simulink model "Ejemplo_1"  (R2022a)
settings: Solver=ode4  StartTime=0.0  StopTime=10.0  FixedStep=0.001  RelTol=1e-3
settings Model: Creator=Anahi Monserrat  LastModifiedBy=Anahi Monserrat

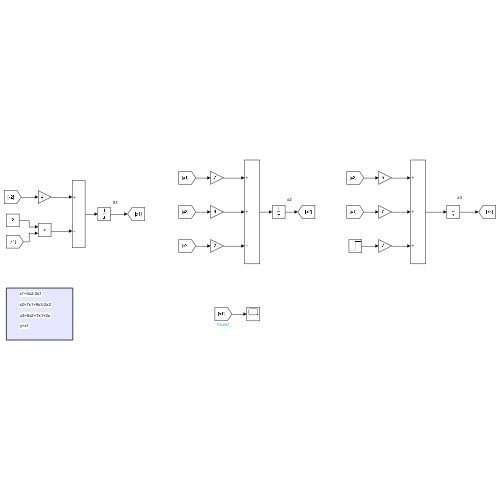
[thumbnail: Simulink's stored preview of the top-level diagram]
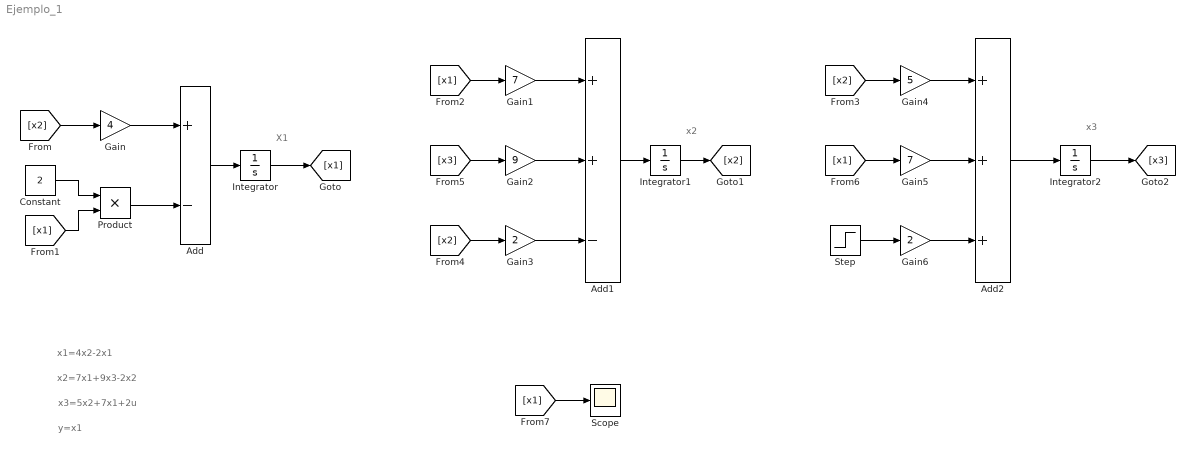
== system Ejemplo_1 ==
  note: y=x1
  note: x3=5x2+7x1+2u
  note: x2=7x1+9x3-2x2
  note: x1=4x2-2x1
  note: x3
  note: x2
  note: X1
  Add : Sum  Inputs=+-
  Add1 : Sum  Inputs=++-
  Add2 : Sum  Inputs=+++
  Constant : Constant  Value=2
  Gain : Gain  Gain=4
  Gain1 : Gain  Gain=7
  Gain2 : Gain  Gain=9
  Gain3 : Gain  Gain=2
  Gain4 : Gain  Gain=5
  Gain5 : Gain  Gain=7
  Gain6 : Gain  Gain=2
  Integrator : Integrator
  Integrator1 : Integrator
  Integrator2 : Integrator
  Product : Product
  Scope : Scope
  Step : Step  SampleTime=0
  wires:
  Add/1 -> Integrator/1
  Gain/1 -> Add/1
  Integrator/1 -> [x1]
  Integrator2/1 -> [x3]
  Integrator1/1 -> [x2]
  [x2] -> Gain/1
  [x1] -> Product/2
  Constant/1 -> Product/1
  Product/1 -> Add/2
  Add1/1 -> Integrator1/1
  [x3] -> Gain2/1
  [x1] -> Gain1/1
  [x2] -> Gain3/1
  Gain3/1 -> Add1/3
  Gain2/1 -> Add1/2
  Gain1/1 -> Add1/1
  Gain4/1 -> Add2/1
  Gain5/1 -> Add2/2
  Gain6/1 -> Add2/3
  [x2] -> Gain4/1
  [x1] -> Gain5/1
  Add2/1 -> Integrator2/1
  Step/1 -> Gain6/1
  [x1] -> Scope/1
